simulink model "single_inverter"  (R2022b)
settings: Solver=ode45  StartTime=0.0  StopTime=0.5  MaxStep=1e-5  MinStep=5e-6  RelTol=1e-3
libraries: spsDiodeLib x8, spsMosfetLib x8, spsSeriesRLCBranchLib x7, spsDCVoltageSourceLib x3, spsVoltageMeasurementLib x3, spsCurrentMeasurementLib x2, powerlib_extras x2, slpidlib x2, spsGroundLib x2, spsLinearTransformerLib x2, simulink x2, spsRMSLib x1
settings Model: Creator=Administrator  LastModifiedBy=Loki

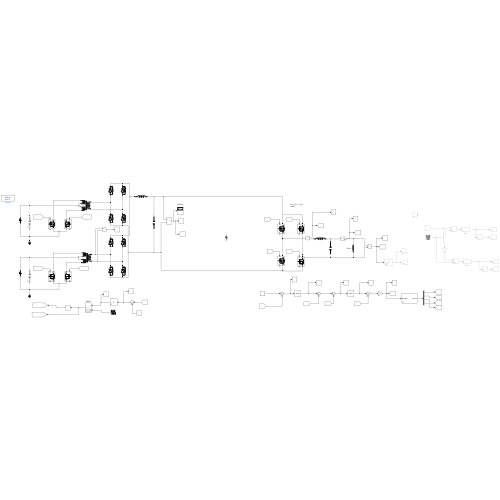
[thumbnail: Simulink's stored preview of the top-level diagram]
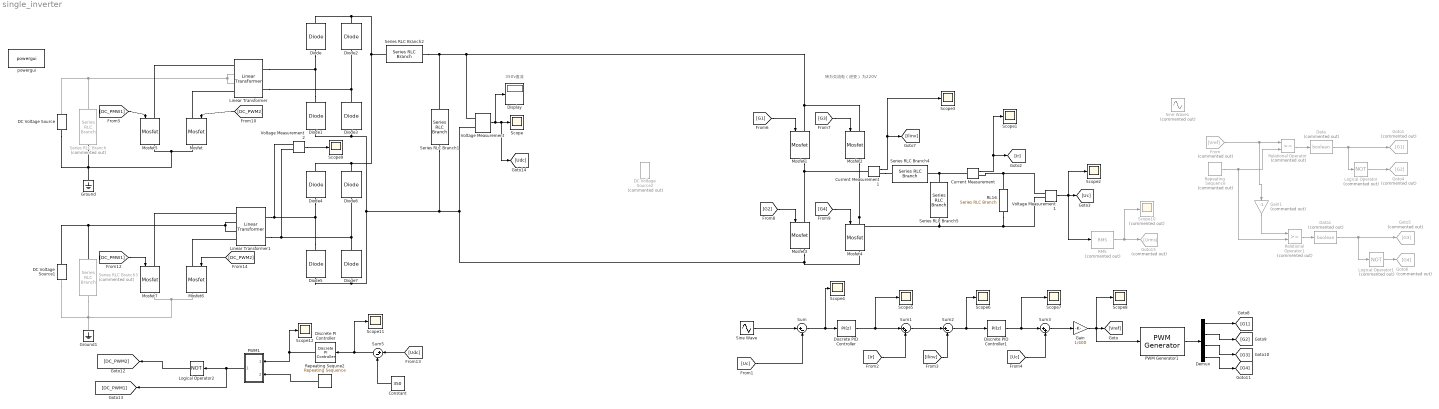
== system single_inverter ==
  note: 转为交流电（逆变）
      | 为220V
  note: 350V直流
  Constant : Constant  Value=350
  Current Measurement : spsCurrentMeasurementLib/Current Measurement  PhasorSimulation=off  OutputType=Complex  PSBequivalent=0
  Current Measurement1 : spsCurrentMeasurementLib/Current Measurement  PhasorSimulation=off  OutputType=Complex  PSBequivalent=0
  DC Voltage Source : spsDCVoltageSourceLib/DC Voltage Source  Amplitude=96  Measurements=None
  DC Voltage Source1 : spsDCVoltageSourceLib/DC Voltage Source  Amplitude=96  Measurements=None
  DC Voltage Source2 : spsDCVoltageSourceLib/DC Voltage Source  Commented=on  Amplitude=350  Measurements=None
  Data : DataTypeConversion  Commented=on  OutDataTypeStr=boolean  SaturateOnIntegerOverflow=off  RndMeth=Floor
  Data1 : DataTypeConversion  Commented=on  OutDataTypeStr=boolean  SaturateOnIntegerOverflow=off  RndMeth=Floor
  Demux : Demux
  Diode{,1..7} (8 alike) : spsDiodeLib/Diode  Ron=0.001  Lon=0  Vf=0.8  IC=0  UseSnubber=0  Rs=500  Cs=250e-9  Measurements=off
  Discrete PI Controller : powerlib_extras/Discrete  Control Blocks/Discrete PI Controller  Kp=2  Ki=50  Par_Limits=[1e6 -1e6]  Init=0  Ts=2e-7
  Discrete PID Controller : slpidlib/PID Controller  Controller=PI  Form=Parallel  TimeDomain=Discrete-time  UseExternalTs=off  SampleTime=-1  IntegratorMethod=Forward Euler  FilterMethod=Forward Euler  ControllerParametersSource=internal  P=0.03115  I=21  UseKiTs=off  D=0  N=100  UseFilter=on  TunerSelectOption=Transfer Function Based (PID Tuner App)  InitialConditionSource=internal  InitialConditionForIntegrator=0  InitialConditionForFilter=0  DifferentiatorICPrevScaledInput=0  ExternalReset=none  TrackingMode=off  Kt=1  LimitOutput=off  SatLimitsSource=internal  UpperSaturationLimit=inf  LowerSaturationLimit=-inf  LinearizeAsGain=off  AntiWindupMode=none  Kb=1  LimitIntegrator=off  UpperIntegratorSaturationLimit=inf  LowerIntegratorSaturationLimit=-inf  POutMin=[]  POutMax=[]  IOutMin=[]  IOutMax=[]  DOutMin=[]  DOutMax=[]  NOutMin=[]  NOutMax=[]  SumOutMin=[]  SumOutMax=[]  SaturationOutMin=[]  SaturationOutMax=[]  PParamMin=[]  PParamMax=[]  IParamMin=[]  IParamMax=[]  DParamMin=[]  DParamMax=[]  NParamMin=[]  NParamMax=[]  KbParamMin=[]  KbParamMax=[]  KtParamMin=[]  KtParamMax=[]  KbOutMin=[]  KbOutMax=[]  KtOutMin=[]  KtOutMax=[]  IntegratorOutMin=[]  IntegratorOutMax=[]  FilterOutMin=[]  FilterOutMax=[]  SumI1OutMin=[]  SumI1OutMax=[]  SumI2OutMin=[]  SumI2OutMax=[]  SumI3OutMin=[]  SumI3OutMax=[]  SumI4OutMin=[]  SumI4OutMax=[]  SumDOutMin=[]  SumDOutMax=[]  DifferentiatorOutMin=[]  DifferentiatorOutMax=[]  FilterDiffOutCoefMin=[]  FilterDiffOutCoefMax=[]  ReciprocalOutMin=[]  ReciprocalOutMax=[]  SumDenOutMin=[]  SumDenOutMax=[]  SumNumOutMin=[]  SumNumOutMax=[]  DivideOutMin=[]  DivideOutMax=[]  UdiffTsProdOutMin=[]  UdiffTsProdOutMax=[]  NTsProdOutMin=[]  NTsProdOutMax=[]  UintegralTsProdOutMin=[]  UintegralTsProdOutMax=[]  UngainTsProdOutMin=[]  UngainTsProdOutMax=[]  ClampingZeroOutDataTypeStr=Inherit: Inherit via back propagation  ClampingZeroOutMin=[]  ClampingZeroOutMax=[]  FilterDenConstantOutDataTypeStr=Inherit: Inherit via back propagation  FilterDenConstantOutMin=[]  FilterDenConstantOutMax=[]  PCopyOutDataTypeStr=Inherit: Inherit via back propagation  PCopyOutMin=[]  PCopyOutMax=[]  NCopyOutDataTypeStr=Inherit: Inherit via back propagation  NCopyOutMin=[]  NCopyOutMax=[]  IntegratorContinuousStateAttributes=''  IntegratorStateMustResolveToSignalObject=off  IntegratorRTWStateStorageClass=Auto  FilterContinuousStateAttributes=''  FilterStateMustResolveToSignalObject=off  FilterRTWStateStorageClass=Auto  ParallelPVariant=InternalParameters  IdealPVariant=Disabled  IVariant=InternalParameters  DVariant=Disabled  IntegratorVariant=Discrete  SatVariant=Disabled  AWVariant=Passthrough  PCopyVariant=Disabled  TRVariant=Disabled  FdbkBlocksVariant=Forward  IdealPFdbkVariant=Disabled  SatFdbkVariant=Disabled  DerivativeFilterVariant=Disabled  NVariant=Disabled  NCopyVariant=Disabled_SignalSpec  FilterICVariant=Disabled  IntegratorICVariant=InternalICs  ExternalResetVariant=Disabled  TRSumVariant=Passthrough  SumFdbkVariant=Disabled  SumVariant=Sum_PI  TsampFilterVariant=InternalTs  TsampNgainVariant=Passthrough  TsampIntegralVariant=Passthrough  ExternalSaturationOutDataTypeStr=Inherit: Same as second input
      settings: LibrarySourceBlock=simulink/Discrete/Discrete PID Controller
  Discrete PID Controller1 : slpidlib/PID Controller  Controller=PI  Form=Parallel  TimeDomain=Discrete-time  UseExternalTs=off  SampleTime=-1  IntegratorMethod=Forward Euler  FilterMethod=Forward Euler  ControllerParametersSource=internal  P=27.066  I=6.67  UseKiTs=off  D=0  N=100  UseFilter=on  TunerSelectOption=Transfer Function Based (PID Tuner App)  InitialConditionSource=internal  InitialConditionForIntegrator=0  InitialConditionForFilter=0  DifferentiatorICPrevScaledInput=0  ExternalReset=none  TrackingMode=off  Kt=1  LimitOutput=off  SatLimitsSource=internal  UpperSaturationLimit=inf  LowerSaturationLimit=-inf  LinearizeAsGain=off  AntiWindupMode=none  Kb=1  LimitIntegrator=off  UpperIntegratorSaturationLimit=inf  LowerIntegratorSaturationLimit=-inf  POutMin=[]  POutMax=[]  IOutMin=[]  IOutMax=[]  DOutMin=[]  DOutMax=[]  NOutMin=[]  NOutMax=[]  SumOutMin=[]  SumOutMax=[]  SaturationOutMin=[]  SaturationOutMax=[]  PParamMin=[]  PParamMax=[]  IParamMin=[]  IParamMax=[]  DParamMin=[]  DParamMax=[]  NParamMin=[]  NParamMax=[]  KbParamMin=[]  KbParamMax=[]  KtParamMin=[]  KtParamMax=[]  KbOutMin=[]  KbOutMax=[]  KtOutMin=[]  KtOutMax=[]  IntegratorOutMin=[]  IntegratorOutMax=[]  FilterOutMin=[]  FilterOutMax=[]  SumI1OutMin=[]  SumI1OutMax=[]  SumI2OutMin=[]  SumI2OutMax=[]  SumI3OutMin=[]  SumI3OutMax=[]  SumI4OutMin=[]  SumI4OutMax=[]  SumDOutMin=[]  SumDOutMax=[]  DifferentiatorOutMin=[]  DifferentiatorOutMax=[]  FilterDiffOutCoefMin=[]  FilterDiffOutCoefMax=[]  ReciprocalOutMin=[]  ReciprocalOutMax=[]  SumDenOutMin=[]  SumDenOutMax=[]  SumNumOutMin=[]  SumNumOutMax=[]  DivideOutMin=[]  DivideOutMax=[]  UdiffTsProdOutMin=[]  UdiffTsProdOutMax=[]  NTsProdOutMin=[]  NTsProdOutMax=[]  UintegralTsProdOutMin=[]  UintegralTsProdOutMax=[]  UngainTsProdOutMin=[]  UngainTsProdOutMax=[]  ClampingZeroOutDataTypeStr=Inherit: Inherit via back propagation  ClampingZeroOutMin=[]  ClampingZeroOutMax=[]  FilterDenConstantOutDataTypeStr=Inherit: Inherit via back propagation  FilterDenConstantOutMin=[]  FilterDenConstantOutMax=[]  PCopyOutDataTypeStr=Inherit: Inherit via back propagation  PCopyOutMin=[]  PCopyOutMax=[]  NCopyOutDataTypeStr=Inherit: Inherit via back propagation  NCopyOutMin=[]  NCopyOutMax=[]  IntegratorContinuousStateAttributes=''  IntegratorStateMustResolveToSignalObject=off  IntegratorRTWStateStorageClass=Auto  FilterContinuousStateAttributes=''  FilterStateMustResolveToSignalObject=off  FilterRTWStateStorageClass=Auto  ParallelPVariant=InternalParameters  IdealPVariant=Disabled  IVariant=InternalParameters  DVariant=Disabled  IntegratorVariant=Discrete  SatVariant=Disabled  AWVariant=Passthrough  PCopyVariant=Disabled  TRVariant=Disabled  FdbkBlocksVariant=Forward  IdealPFdbkVariant=Disabled  SatFdbkVariant=Disabled  DerivativeFilterVariant=Disabled  NVariant=Disabled  NCopyVariant=Disabled_SignalSpec  FilterICVariant=Disabled  IntegratorICVariant=InternalICs  ExternalResetVariant=Disabled  TRSumVariant=Passthrough  SumFdbkVariant=Disabled  SumVariant=Sum_PI  TsampFilterVariant=InternalTs  TsampNgainVariant=Passthrough  TsampIntegralVariant=Passthrough  ExternalSaturationOutDataTypeStr=Inherit: Same as second input
      settings: LibrarySourceBlock=simulink/Discrete/Discrete PID Controller
  Display : Display
  From : From  Commented=on  GotoTag=Vref
  Gain : Gain  Gain=1/400
  Gain1 : Gain  Commented=on  Gain=-1
  Goto1 : Goto  Commented=on  GotoTag=G1
  Goto15 : Goto  Commented=on  GotoTag=Urms
  Goto4 : Goto  Commented=on  GotoTag=G2
  Goto5 : Goto  Commented=on  GotoTag=G3
  Goto6 : Goto  Commented=on  GotoTag=G4
  Ground : spsGroundLib/Ground  LConnTagsString=a
  Ground1 : spsGroundLib/Ground  LConnTagsString=a
  Linear Transformer : spsLinearTransformerLib/Linear Transformer  UNITS=SI  NominalPower=[ 3000 60 ]  winding1=[96 0 1e-6]  winding2=[96 0 1e-6]  ThreeWindings=on  winding3=[24 0 5e-6]  RmLm=[1.0804e+06 2866]  Measurements=None  DataType=on
  Linear Transformer1 : spsLinearTransformerLib/Linear Transformer  UNITS=SI  NominalPower=[ 3000 60 ]  winding1=[96 0 1e-6]  winding2=[96 0 1e-6]  ThreeWindings=on  winding3=[24 0 5e-6]  RmLm=[1.0804e+06 2866]  Measurements=None  DataType=on
  Logical Operator : Logic  Commented=on  Operator=NOT  AllPortsSameDT=off  OutDataTypeStr=boolean
  Logical Operator1 : Logic  Commented=on  Operator=NOT  AllPortsSameDT=off  OutDataTypeStr=boolean
  Logical Operator2 : Logic  Operator=NOT  AllPortsSameDT=off  OutDataTypeStr=boolean
  Mosfet{,1..7} (8 alike) : spsMosfetLib/Mosfet  Ron=0.1  Lon=0  Rd=0.01  Vfd=0  IC=0  Rs=1e5  Cs=inf  Measurements=on
  PWM Generator1 : powerlib_extras/Control  Blocks/PWM Generator  GeneratorMode="2-arm  bridge (4 pulses)"  Fc=10000  Internal=off  mIndex=0.4  Freq=60  Phase=0
      link override Triangle: rep_seq_y=[0 -1 1 0]
  PWM1 : Subsystem
  RL16 : spsSeriesRLCBranchLib/Series RLC Branch  LConnTagsString=__new0  RConnTagsString=__new0  BranchType=R  Resistance=50  Inductance=1e-3  SetiL0=off  InitialCurrent=0  Capacitance=3000e-6  Setx0=off  InitialVoltage=0  Measurements=None
  RMS : spsRMSLib/RMS  Commented=on  TrueRMS=on  Freq=50  RMSInit=0  Ts=0
  Relational Operator : RelationalOperator  Commented=on  OutDataTypeStr=boolean  RndMeth=Simplest  InputSameDT=off
  Relational Operator1 : RelationalOperator  Commented=on  OutDataTypeStr=boolean  RndMeth=Simplest  InputSameDT=off
  Repeating Sequence : simulink/Sources/Repeating Sequence  Commented=on  rep_seq_t=[0 1/20000 1/10000]  rep_seq_y=[-1 1 -1]
  Repeating Sequne2 : simulink/Sources/Repeating Sequence  rep_seq_t=[0 5e-6 10e-6 15e-6 20e-6]  rep_seq_y=[0 1 0 -1 0]
  Scope{,1..9,11..12} (12 alike) : Scope
  Scope10 : Scope  Commented=on
  Series RLC Branch : spsSeriesRLCBranchLib/Series RLC Branch  Commented=on  LConnTagsString=__new0  RConnTagsString=__new0  BranchType=C  Resistance=1  Inductance=1e-3  SetiL0=off  InitialCurrent=0  Capacitance=1e-6  Setx0=off  InitialVoltage=0  Measurements=None
  Series RLC Branch1 : spsSeriesRLCBranchLib/Series RLC Branch  LConnTagsString=__new0  RConnTagsString=__new0  BranchType=C  Resistance=1  Inductance=1e-3  SetiL0=off  InitialCurrent=0  Capacitance=500e-6  Setx0=off  InitialVoltage=0  Measurements=None
  Series RLC Branch2 : spsSeriesRLCBranchLib/Series RLC Branch  LConnTagsString=__new0  RConnTagsString=__new0  BranchType=L  Resistance=1  Inductance=2e-3  SetiL0=off  InitialCurrent=0  Capacitance=1e-6  Setx0=off  InitialVoltage=0  Measurements=None
  Series RLC Branch3 : spsSeriesRLCBranchLib/Series RLC Branch  Commented=on  LConnTagsString=__new0  RConnTagsString=__new0  BranchType=C  Resistance=1  Inductance=1e-3  SetiL0=off  InitialCurrent=0  Capacitance=1e-6  Setx0=off  InitialVoltage=0  Measurements=None
  Series RLC Branch4 : spsSeriesRLCBranchLib/Series RLC Branch  LConnTagsString=__new0  RConnTagsString=__new0  BranchType=L  Resistance=0  Inductance=4.06e-3  SetiL0=off  InitialCurrent=0  Capacitance=1e-6  Setx0=off  InitialVoltage=0  Measurements=None
  Series RLC Branch5 : spsSeriesRLCBranchLib/Series RLC Branch  LConnTagsString=__new0  RConnTagsString=__new0  BranchType=C  Resistance=1  Inductance=1e-3  SetiL0=off  InitialCurrent=0  Capacitance=6.23e-6  Setx0=off  InitialVoltage=0  Measurements=None
  Sine Wave : Sin  Amplitude=311  Frequency=100*pi  SampleTime=0
  Sine Wave1 : Sin  Commented=on  Amplitude=0.98  Frequency=100*pi  SampleTime=0
  Sum : Sum  Inputs=|+-
  Sum1 : Sum  Inputs=|++
  Sum2 : Sum  Inputs=|+-
  Sum3 : Sum  Inputs=|++
  Sum5 : Sum  Inputs=|+-
  Voltage Measurement : spsVoltageMeasurementLib/Voltage Measurement  PhasorSimulation=off  OutputType=Complex  PSBequivalent=0
  Voltage Measurement1 : spsVoltageMeasurementLib/Voltage Measurement  PhasorSimulation=off  OutputType=Complex  PSBequivalent=0
  Voltage Measurement2 : spsVoltageMeasurementLib/Voltage Measurement  PhasorSimulation=off  OutputType=Complex  PSBequivalent=0
  powergui : spspowerguiLib/powergui  Priority=1  SimulationMode=Discrete  SampleTime=5e-7  frequency=60  Iterations=50  frequencyindice=0  Pbase=100e6  ErrMax=1e-4  UnitsV=kV  UnitsW=MW  buscounter=0  FunctionMessages=off  echomessages=off  EnableUseOfTLC=off  CurrentSourceSwitches=off  DisableSnubberDevices=off  DisableRonSwitches=off  DisableVfSwitches=off  DisplayEquations=off  AutomaticDiscreteSolvers=off  SolverType=Tustin/Backward Euler (TBE)  Interpol=off  ExternalGateDelay=off  methode=off  Ts=100  x0status=blocks  SPID=on  SwTol=0  HookPort=off  NonlinearTolerance=1e-4  nMaxIteration=100  ContinueOnMaxIteration=off  RestoreLinks=warning  ResistiveCurrentMeasurement=off  Frange=[0:2:500]  Ylog=off  Xlog=on  ShowGrid=off  save=off  variable=ZData  structure=0  ZoomFFT=off  StartTime=0.0  cycles=1  DisplayStyle=1  fundamental=60  FreqAxis=off  MaxFrequency=1000  frequencyindicesteady=1  RmsSteady=1  display=off
  wires:
  Current Measurement/1 -> Scope1/1, [Ir]
  [G4] -> Mosfet4/1
  [G2] -> Mosfet3/1
  Voltage Measurement1/1 -> RMS/1, Scope2/1, [Uc]
  [G3] -> Mosfet2/1
  [G1] -> Mosfet1/1
  Sine Wave/1 -> Sum/1
  Sum/1 -> Scope4/1, Discrete PID Controller/1
  Sum1/1 -> Sum2/1
  Sum2/1 -> Scope6/1, Discrete PID Controller1/1
  Discrete PID Controller1/1 -> Scope7/1, Sum3/1
  Sum3/1 -> Gain/1
  Gain/1 -> PWM Generator1/1, Scope8/1, [Vref]
  From/1 -> Gain1/1, Relational Operator/1
  Repeating Sequence/1 -> Relational Operator1/2, Relational Operator/2
  Logical Operator/1 -> Goto4/1
  Logical Operator1/1 -> Goto6/1
  Gain1/1 -> Relational Operator1/1
  [Uc] -> Sum/2
  [Ir] -> Sum1/2
  Current Measurement1/1 -> Scope3/1, [Ilinv]
  [Ilinv] -> Sum2/2
  [Uc] -> Sum3/2
  Discrete PID Controller/1 -> Scope5/1, Sum1/1
  Relational Operator/1 -> Data/1
  Data/1 -> Logical Operator/1, Goto1/1
  Relational Operator1/1 -> Data1/1
  Data1/1 -> Logical Operator1/1, Goto5/1
  PWM Generator1/1 -> Demux/1
  Demux/1 -> [G1]
  Demux/2 -> [G2]
  Demux/3 -> [G3]
  Demux/4 -> [G4]
  Sum5/1 -> Scope11/1, Discrete PI Controller/1
  [Udc] -> Sum5/1
  Constant/1 -> Sum5/2
  Repeating Sequne2/1 -> PWM1/2(In2)
  PWM1/1(Out1) -> [DC_PWM1], Logical Operator2/1
  Logical Operator2/1 -> [DC_PWM2]
  Discrete PI Controller/1 -> Scope12/1, PWM1/1(In1)
  Voltage Measurement/1 -> Display/1, [Udc], Scope/1
  [DC_PMW1] -> Mosfet5/1
  [DC_PMW1] -> Mosfet7/1
  [DC_PWM2] -> Mosfet/1
  [DC_PWM2] -> Mosfet6/1
  Voltage Measurement2/1 -> Scope9/1
  RMS/1 -> Scope10/1, Goto15/1
  connections:
  Voltage Measurement1/LConn1 -- Current Measurement/RConn1 -- RL16/LConn1
  Series RLC Branch4/LConn1 -- Series RLC Branch5/LConn1 -- Current Measurement/LConn1
  Series RLC Branch5/RConn1 -- Voltage Measurement1/LConn2 -- RL16/RConn1 -- Mosfet2/RConn1 -- Mosfet4/LConn1
  Mosfet3/RConn1 -- Series RLC Branch1/RConn1 -- Diode5/LConn1 -- Diode7/LConn1 -- Diode1/LConn1 -- Diode3/LConn1 -- Voltage Measurement/LConn2 -- Mosfet4/RConn1
  Current Measurement1/LConn1 -- Mosfet3/LConn1 -- Mosfet1/RConn1
  Current Measurement1/RConn1 -- Series RLC Branch4/RConn1
  Mosfet5/RConn1 -- Mosfet/RConn1 -- Ground/LConn1 -- Series RLC Branch/RConn1 -- DC Voltage Source/LConn1
  Diode2/LConn1 -- Diode3/RConn1 -- Linear Transformer/LConn2
  Series RLC Branch3/LConn1 -- DC Voltage Source1/RConn1 -- Linear Transformer1/RConn3 -- Linear Transformer1/RConn2
  Series RLC Branch2/RConn1 -- Diode4/RConn1 -- Diode6/RConn1 -- Diode/RConn1 -- Diode2/RConn1
  Diode5/RConn1 -- Voltage Measurement2/LConn1 -- Linear Transformer1/LConn1 -- Diode4/LConn1
  Series RLC Branch/LConn1 -- Linear Transformer/RConn3 -- Linear Transformer/RConn2 -- DC Voltage Source/RConn1
  Series RLC Branch3/RConn1 -- DC Voltage Source1/LConn1 -- Ground1/LConn1 -- Mosfet7/RConn1 -- Mosfet6/RConn1
  Diode1/RConn1 -- Diode/LConn1 -- Linear Transformer/LConn1
  Diode6/LConn1 -- Voltage Measurement2/LConn2 -- Linear Transformer1/LConn2 -- Diode7/RConn1
  Mosfet5/LConn1 -- Linear Transformer/RConn1
  Linear Transformer1/RConn4 -- Mosfet6/LConn1
  Linear Transformer1/RConn1 -- Mosfet7/LConn1
  Mosfet/LConn1 -- Linear Transformer/RConn4
  Series RLC Branch2/LConn1 -- Mosfet2/LConn1 -- Mosfet1/LConn1 -- Voltage Measurement/LConn1 -- Series RLC Branch1/LConn1

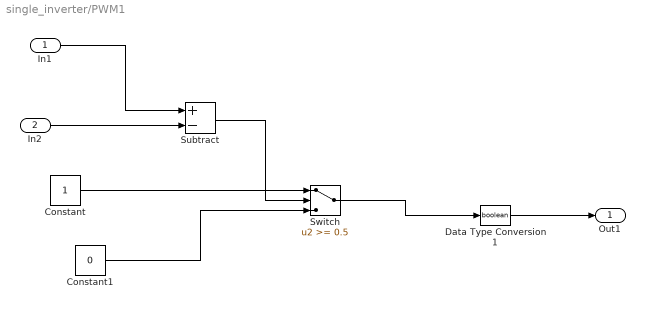
== system single_inverter/PWM1 ==
  In1 : Inport
  In2 : Inport  Port=2
  Constant : Constant
  Constant1 : Constant  Value=0
  Data Type Conversion1 : DataTypeConversion  OutDataTypeStr=boolean
  Subtract : Sum  Inputs=+-
  Switch : Switch  Threshold=0.5  SaturateOnIntegerOverflow=off  InputSameDT=off
  Out1 : Outport
  wires:
  Constant/1 -> Switch/1
  Subtract/1 -> Switch/2
  In2/1 -> Subtract/2
  In1/1 -> Subtract/1
  Switch/1 -> Data Type Conversion1/1
  Data Type Conversion1/1 -> Out1/1
  Constant1/1 -> Switch/3
